simulink model "EvReferenceApplication"  (R2024a)
settings: Solver=daessc  StartTime=0  StopTime=2474  FixedStep=0.01  RelTol=1e-3
undefined symbols (not defined in the file or in its folder): anomaly_start, bat_temp_init, battery, driver_reaction, ext_wind, pipe, pump, pump_speed, radiator, sim_time, SRE, T_set, tank, valve
libraries: fl_lib x139, LiBatteryElements_lib x16, nesl_utility x14, SimscapeFluids_lib x7, autolibshared x2, simulink x1, autolibutils x1, slpidlib x1, simulink_extras x1
(part 3 of 4)

== system EvReferenceApplication/Passenger Car/Electric Plant/Powertrain Blockset/Motor ==
  MotTrqCmd : Inport
  MotSpd : Inport  Port=2
  BusVolt : Inport  Port=3
  MotGenEvDynamic : ModelReference  ModelNameDialog=MotGenEvDynamic.slx  SimulationMode=Normal  VariantControl=MotGenEvDynamic  ModelReferenceVersion=10.1
  MotGenEvMapped : ModelReference  ModelNameDialog=MotGenEvMapped.slx  SimulationMode=Normal  VariantControl=MotGenEvMapped  ModelReferenceVersion=8.3
  MotTrq : Outport  VectorParamsAs1DForOutWhenUnconnected=off
  MotCurnt : Outport  Port=2  VectorParamsAs1DForOutWhenUnconnected=off

== system EvReferenceApplication/Passenger Car/Electric Plant/Powertrain Blockset/Subsystem2 ==
  In Bus Element : Inport  PortName=BMS_Info  Element=SOC
  Bus Selector : BusSelector  OutputSignals=SOC_CC
  Data Type Conversion : DataTypeConversion  SaturateOnIntegerOverflow=off  RndMeth=Floor
  Rate Transition : RateTransition  Commented=through
  convert2percent : Gain  Gain=100
  BattSOC : Outport
  wires:
  In Bus Element/1 -> Bus Selector/1
  convert2percent/1 -> Data Type Conversion/1
  Bus Selector/1 -> convert2percent/1  "<SOC_CC>"
  Data Type Conversion/1 -> Rate Transition/1
  Rate Transition/1 -> BattSOC/1

== system EvReferenceApplication/Passenger Car/Electric Plant/Powertrain Blockset/Temp Selection ==
  AmbTmp : Inport
  Constant : Constant  Value=bat_temp_init
  Convert degC to K : Subsystem
  Manual Switch : ManualSwitch  CurrentSetting=0
  BattTmp : Outport
  wires:
  AmbTmp/1 -> Manual Switch/1
  Manual Switch/1 -> BattTmp/1
  Convert degC to K/1(Out1) -> Manual Switch/2
  Constant/1 -> Convert degC to K/1(In1)

== system EvReferenceApplication/Passenger Car/Electric Plant/Powertrain Blockset/BMS Signal Creation/Convert K to degC ==
  In1 : Inport
  Constant1 : Constant  Value=273.15
  Sum : Sum  Inputs=+-
  Out1 : Outport
  wires:
  In1/1 -> Sum/1
  Constant1/1 -> Sum/2
  Sum/1 -> Out1/1

== system EvReferenceApplication/Passenger Car/Electric Plant/Powertrain Blockset/Battery Cooling/Air Stream ==
  V : Inport
  Air density [kg/m^3] : Constant  Value=1.225
  Air velocity [m/s] : Bias  Bias=5  SaturateOnIntegerOverflow=off
  Product : Product  Inputs=3
  Radiator area [m^2] : Constant  Value=radiator.area_air
  Simulink-PS Converter1 : nesl_utility/Simulink-PS Converter  PhysicalDomain=network_engine_domain  SubClassName=ps_input  LeftPortType=input  RightPortType=output  PseudoPeriodic=off  Frequencies=[]  NoiseDistribution=none  NoiseParameters=[]  Unit=kg/s  AffineConversion=off  FilteringAndDerivatives=filter  SimscapeFilterOrder=1  InputFilterTimeConstant=0.01  UdotUserProvided=0
  mdot : PMIOPort  Side=Right
  wires:
  V/1 -> Air velocity [m/s]/1
  Product/1 -> Simulink-PS Converter1/1
  Radiator area [m^2]/1 -> Product/2
  Air density [kg/m^3]/1 -> Product/3
  Air velocity [m/s]/1 -> Product/1
  connections:
  mdot/RConn1 -- Simulink-PS Converter1/RConn1

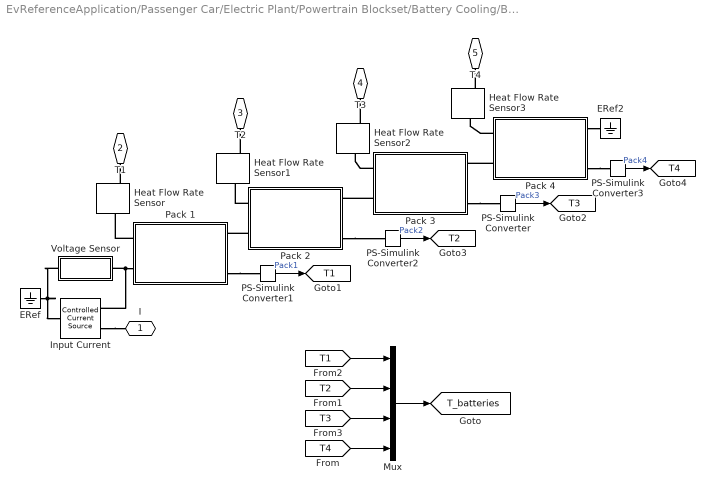
== system EvReferenceApplication/Passenger Car/Electric Plant/Powertrain Blockset/Battery Cooling/Battery1 ==
  ERef : fl_lib/Electrical/Electrical Elements/Electrical Reference
  ERef2 : fl_lib/Electrical/Electrical Elements/Electrical Reference
  Heat Flow Rate Sensor{,1..3} (4 alike) : fl_lib/Thermal/Thermal Sensors/Heat Flow Rate Sensor
  Input Current : fl_lib/Electrical/Electrical Sources/Controlled Current Source
  Mux : Mux
  PS-Simulink Converter{,1..3} (4 alike) : nesl_utility/PS-Simulink Converter  PhysicalDomain=network_engine_domain  SubClassName=ps_output  LeftPortType=input  RightPortType=output  PseudoPeriodic=off  Frequencies=[]  VectorFormat=1-D array  Unit=degC  AffineConversion=on
  Pack 1 : Subsystem  Tag=PublishSubsystem  mask(Lithium cell (one RC-branch equivalent circuit)){Ncells=battery.NCell, Qe_init=battery.Qe_init, T_init=bat_temp_init+273.15, Capacity_LUT=battery.capacity_LUT, Em_LUT=battery.Em_LUT, R0_LUT=battery.R0_LUT, R1_LUT=battery.R1_LUT, C1_LUT=battery.C1_LUT, cell_mass=battery.cell_mass, cell_Cp_heat=battery.cell_Cp, SOC_LUT=battery.SOC_LUT, Temperature_LUT=battery.temperature_LUT}
      mask prompts: Ncells "Number of series-connected cells"; Qe_init "Initial cell charge deficit (A*hr)"; T_init "Initial cell temperature (K)"; Capacity_LUT "Capacity (A*hr, 1xN table)"; Em_LUT "Em open-circuit voltage, Em (volts, MxN table)"; R0_LUT "R0 terminal resistance (ohms, MxN table)"; R1_LUT "R1 cell resistance (ohms, MxN table)"; C1_LUT "C1 capacitance (farads, MxN table)"; cell_mass "Cell mass (kg)"; cell_Cp_heat "Cell specific heat (J/kg/K)"; SOC_LUT "SOC table breakpoints (Mx1 array)"; Temperature_LUT "Temperature table breakpoints (K, 1xN array)"
      mask DialogControl ParameterTabVar0 Prompt: Main
      mask DialogControl ParameterTabVar01 Prompt: Electrical (per cell)
      mask DialogControl ParameterTabVar012 Prompt: Thermal (per cell)
      mask DialogControl ParameterTabVar0123 Prompt: Table Breakpoints
      mask Display:
      | % Battery icon
      | plot([2.5 1.3],[0 0])
      | plot([-0.6 -1.6 -1.6 -2.5],[0 0 -0.8 -0.8])
      | patch([1 1 -1 -1]*0.15+1.3,[-1 1 1 -1]*0.4,[0;0;0]);
      | patch([1 1 -1 -1]*0.15+0.0,[-1 1 1 -1]*0.4,[0;0;0]);
      | patch([1 1 -1 -1]*0.15+0.7,[-1 1 1 -1]*0.8,[0;0;0]);
      | patch([1 1 -1 -1]*0.15-0.6,[-1 1 1 -1]*0.8,[0;0;0]);
      | % Thermal port
      | plot([-1.6,-1.3],[1.2,1.2])
      | plot([-1.6,-1.3],[0.5,0.5])
      | plot([-1.6,-2.5],[0.8,0.8])
      | plot(0.2*sin(0:2*pi/50:2*pi)-1.6,0.35*cos(0:2*pi/50:2*pi)+0.85)
      | plot(0.2*sin(0:2*pi/50:pi)-1.3,0.35*cos(0:2*pi/50:pi)+0.85)
      | 
      | % Plot points to set plot range
      | color('white');plot(2.5,1.5);plot(-2.5,-1.5)
      | 
      | color('red')
      | port_label('LConn',1,'H')
      | port_label('LConn',2,'+')
      | port_label('RConn',1,'-')
      | port_label('RConn',2,'SOC')
      | port_label('RConn',3,'T')
  Pack 2 : Subsystem  Tag=PublishSubsystem  mask(Lithium cell (one RC-branch equivalent circuit)){Ncells=battery.NCell, Qe_init=battery.Qe_init, T_init=bat_temp_init+273.15, Capacity_LUT=battery.capacity_LUT, Em_LUT=battery.Em_LUT, R0_LUT=battery.R0_LUT, R1_LUT=battery.R1_LUT, C1_LUT=battery.C1_LUT, cell_mass=battery.cell_mass, cell_Cp_heat=battery.cell_Cp, SOC_LUT=battery.SOC_LUT, Temperature_LUT=battery.temperature_LUT}
      mask prompts: Ncells "Number of series-connected cells"; Qe_init "Initial cell charge deficit (A*hr)"; T_init "Initial cell temperature (K)"; Capacity_LUT "Capacity (A*hr, 1xN table)"; Em_LUT "Em open-circuit voltage, Em (volts, MxN table)"; R0_LUT "R0 terminal resistance (ohms, MxN table)"; R1_LUT "R1 cell resistance (ohms, MxN table)"; C1_LUT "C1 capacitance (farads, MxN table)"; cell_mass "Cell mass (kg)"; cell_Cp_heat "Cell specific heat (J/kg/K)"; SOC_LUT "SOC table breakpoints (Mx1 array)"; Temperature_LUT "Temperature table breakpoints (K, 1xN array)"
      mask DialogControl ParameterTabVar0 Prompt: Main
      mask DialogControl ParameterTabVar01 Prompt: Electrical (per cell)
      mask DialogControl ParameterTabVar012 Prompt: Thermal (per cell)
      mask DialogControl ParameterTabVar0123 Prompt: Table Breakpoints
      mask Display:
      | % Battery icon
      | plot([2.5 1.3],[0 0])
      | plot([-0.6 -1.6 -1.6 -2.5],[0 0 -0.8 -0.8])
      | patch([1 1 -1 -1]*0.15+1.3,[-1 1 1 -1]*0.4,[0;0;0]);
      | patch([1 1 -1 -1]*0.15+0.0,[-1 1 1 -1]*0.4,[0;0;0]);
      | patch([1 1 -1 -1]*0.15+0.7,[-1 1 1 -1]*0.8,[0;0;0]);
      | patch([1 1 -1 -1]*0.15-0.6,[-1 1 1 -1]*0.8,[0;0;0]);
      | % Thermal port
      | plot([-1.6,-1.3],[1.2,1.2])
      | plot([-1.6,-1.3],[0.5,0.5])
      | plot([-1.6,-2.5],[0.8,0.8])
      | plot(0.2*sin(0:2*pi/50:2*pi)-1.6,0.35*cos(0:2*pi/50:2*pi)+0.85)
      | plot(0.2*sin(0:2*pi/50:pi)-1.3,0.35*cos(0:2*pi/50:pi)+0.85)
      | 
      | % Plot points to set plot range
      | color('white');plot(2.5,1.5);plot(-2.5,-1.5)
      | 
      | color('red')
      | port_label('LConn',1,'H')
      | port_label('LConn',2,'+')
      | port_label('RConn',1,'-')
      | port_label('RConn',2,'SOC')
      | port_label('RConn',3,'T')
  Pack 3 : Subsystem  Tag=PublishSubsystem  mask(Lithium cell (one RC-branch equivalent circuit)){Ncells=battery.NCell, Qe_init=battery.Qe_init, T_init=bat_temp_init+273.15, Capacity_LUT=battery.capacity_LUT, Em_LUT=battery.Em_LUT, R0_LUT=battery.R0_LUT, R1_LUT=battery.R1_LUT, C1_LUT=battery.C1_LUT, cell_mass=battery.cell_mass, cell_Cp_heat=battery.cell_Cp, SOC_LUT=battery.SOC_LUT, Temperature_LUT=battery.temperature_LUT}
      mask prompts: Ncells "Number of series-connected cells"; Qe_init "Initial cell charge deficit (A*hr)"; T_init "Initial cell temperature (K)"; Capacity_LUT "Capacity (A*hr, 1xN table)"; Em_LUT "Em open-circuit voltage, Em (volts, MxN table)"; R0_LUT "R0 terminal resistance (ohms, MxN table)"; R1_LUT "R1 cell resistance (ohms, MxN table)"; C1_LUT "C1 capacitance (farads, MxN table)"; cell_mass "Cell mass (kg)"; cell_Cp_heat "Cell specific heat (J/kg/K)"; SOC_LUT "SOC table breakpoints (Mx1 array)"; Temperature_LUT "Temperature table breakpoints (K, 1xN array)"
      mask DialogControl ParameterTabVar0 Prompt: Main
      mask DialogControl ParameterTabVar01 Prompt: Electrical (per cell)
      mask DialogControl ParameterTabVar012 Prompt: Thermal (per cell)
      mask DialogControl ParameterTabVar0123 Prompt: Table Breakpoints
      mask Display:
      | % Battery icon
      | plot([2.5 1.3],[0 0])
      | plot([-0.6 -1.6 -1.6 -2.5],[0 0 -0.8 -0.8])
      | patch([1 1 -1 -1]*0.15+1.3,[-1 1 1 -1]*0.4,[0;0;0]);
      | patch([1 1 -1 -1]*0.15+0.0,[-1 1 1 -1]*0.4,[0;0;0]);
      | patch([1 1 -1 -1]*0.15+0.7,[-1 1 1 -1]*0.8,[0;0;0]);
      | patch([1 1 -1 -1]*0.15-0.6,[-1 1 1 -1]*0.8,[0;0;0]);
      | % Thermal port
      | plot([-1.6,-1.3],[1.2,1.2])
      | plot([-1.6,-1.3],[0.5,0.5])
      | plot([-1.6,-2.5],[0.8,0.8])
      | plot(0.2*sin(0:2*pi/50:2*pi)-1.6,0.35*cos(0:2*pi/50:2*pi)+0.85)
      | plot(0.2*sin(0:2*pi/50:pi)-1.3,0.35*cos(0:2*pi/50:pi)+0.85)
      | 
      | % Plot points to set plot range
      | color('white');plot(2.5,1.5);plot(-2.5,-1.5)
      | 
      | color('red')
      | port_label('LConn',1,'H')
      | port_label('LConn',2,'+')
      | port_label('RConn',1,'-')
      | port_label('RConn',2,'SOC')
      | port_label('RConn',3,'T')
  Pack 4 : Subsystem  Tag=PublishSubsystem  mask(Lithium cell (one RC-branch equivalent circuit)){Ncells=battery.NCell, Qe_init=battery.Qe_init, T_init=bat_temp_init+273.15, Capacity_LUT=battery.capacity_LUT, Em_LUT=battery.Em_LUT, R0_LUT=battery.R0_LUT, R1_LUT=battery.R1_LUT, C1_LUT=battery.C1_LUT, cell_mass=battery.cell_mass, cell_Cp_heat=battery.cell_Cp, SOC_LUT=battery.SOC_LUT, Temperature_LUT=battery.temperature_LUT}
      mask prompts: Ncells "Number of series-connected cells"; Qe_init "Initial cell charge deficit (A*hr)"; T_init "Initial cell temperature (K)"; Capacity_LUT "Capacity (A*hr, 1xN table)"; Em_LUT "Em open-circuit voltage, Em (volts, MxN table)"; R0_LUT "R0 terminal resistance (ohms, MxN table)"; R1_LUT "R1 cell resistance (ohms, MxN table)"; C1_LUT "C1 capacitance (farads, MxN table)"; cell_mass "Cell mass (kg)"; cell_Cp_heat "Cell specific heat (J/kg/K)"; SOC_LUT "SOC table breakpoints (Mx1 array)"; Temperature_LUT "Temperature table breakpoints (K, 1xN array)"
      mask DialogControl ParameterTabVar0 Prompt: Main
      mask DialogControl ParameterTabVar01 Prompt: Electrical (per cell)
      mask DialogControl ParameterTabVar012 Prompt: Thermal (per cell)
      mask DialogControl ParameterTabVar0123 Prompt: Table Breakpoints
      mask Display:
      | % Battery icon
      | plot([2.5 1.3],[0 0])
      | plot([-0.6 -1.6 -1.6 -2.5],[0 0 -0.8 -0.8])
      | patch([1 1 -1 -1]*0.15+1.3,[-1 1 1 -1]*0.4,[0;0;0]);
      | patch([1 1 -1 -1]*0.15+0.0,[-1 1 1 -1]*0.4,[0;0;0]);
      | patch([1 1 -1 -1]*0.15+0.7,[-1 1 1 -1]*0.8,[0;0;0]);
      | patch([1 1 -1 -1]*0.15-0.6,[-1 1 1 -1]*0.8,[0;0;0]);
      | % Thermal port
      | plot([-1.6,-1.3],[1.2,1.2])
      | plot([-1.6,-1.3],[0.5,0.5])
      | plot([-1.6,-2.5],[0.8,0.8])
      | plot(0.2*sin(0:2*pi/50:2*pi)-1.6,0.35*cos(0:2*pi/50:2*pi)+0.85)
      | plot(0.2*sin(0:2*pi/50:pi)-1.3,0.35*cos(0:2*pi/50:pi)+0.85)
      | 
      | % Plot points to set plot range
      | color('white');plot(2.5,1.5);plot(-2.5,-1.5)
      | 
      | color('red')
      | port_label('LConn',1,'H')
      | port_label('LConn',2,'+')
      | port_label('RConn',1,'-')
      | port_label('RConn',2,'SOC')
      | port_label('RConn',3,'T')
  Voltage Sensor : Subsystem
      mask Display: disp('V_load')
  I : PMIOPort  Side=Left
  T1 : PMIOPort  Port=2  Side=Right
  T2 : PMIOPort  Port=3  Side=Right
  T3 : PMIOPort  Port=4  Side=Right
  T4 : PMIOPort  Port=5  Side=Right
  tag scope: T1=global, T2=global, T3=global, T4=global, T_batteries=global
  wires:
  PS-Simulink Converter/1 -> [T3]  "Pack3"
  PS-Simulink Converter2/1 -> [T2]  "Pack2"
  PS-Simulink Converter3/1 -> [T4]  "Pack4"
  [T1] -> Mux/1
  [T2] -> Mux/2
  [T3] -> Mux/3
  [T4] -> Mux/4
  Mux/1 -> [T_batteries]
  PS-Simulink Converter1/1 -> [T1]  "Pack1"
  connections:
  Pack 3/LConn2 -- Pack 2/RConn1
  Pack 3/RConn3 -- PS-Simulink Converter/LConn1
  Voltage Sensor/LConn1 -- Pack 1/LConn2 -- Input Current/RConn2
  Pack 2/LConn2 -- Pack 1/RConn1
  Pack 4/RConn1 -- ERef2/LConn1
  Input Current/RConn1 -- I/RConn1
  Voltage Sensor/RConn1 -- ERef/LConn1 -- Input Current/LConn1
  Pack 4/LConn2 -- Pack 3/RConn1
  Pack 2/RConn3 -- PS-Simulink Converter2/LConn1
  Pack 4/RConn3 -- PS-Simulink Converter3/LConn1
  Pack 1/RConn3 -- PS-Simulink Converter1/LConn1
  Pack 1/LConn1 -- Heat Flow Rate Sensor/LConn1
  Heat Flow Rate Sensor/RConn2 -- T1/RConn1
  Heat Flow Rate Sensor1/RConn2 -- T2/RConn1
  Pack 2/LConn1 -- Heat Flow Rate Sensor1/LConn1
  Heat Flow Rate Sensor2/RConn2 -- T3/RConn1
  Pack 3/LConn1 -- Heat Flow Rate Sensor2/LConn1
  Heat Flow Rate Sensor3/RConn2 -- T4/RConn1
  Pack 4/LConn1 -- Heat Flow Rate Sensor3/LConn1

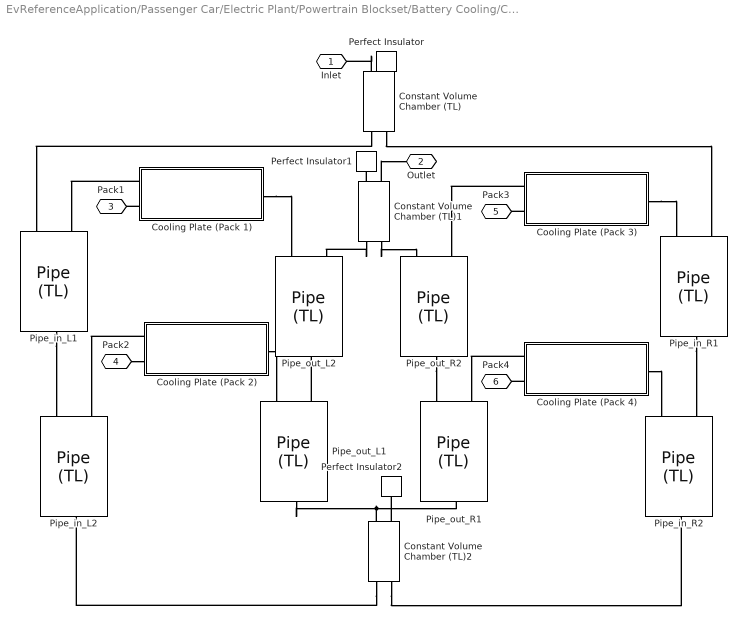
== system EvReferenceApplication/Passenger Car/Electric Plant/Powertrain Blockset/Battery Cooling/Cold Plate ==
  Constant Volume Chamber (TL) : fl_lib/Thermal Liquid/Elements/Constant Volume Chamber (TL)  volume=0.001 m^3  num_ports=foundation.enum.num_ports.three  area_A=3 cm^2  area_B=3 cm^2  area_C=3 cm^2  area_D=0.01 m^2  p_I_specify=off  p_I_priority=High  p_I=0.101325 MPa  p_I_nominal_specify=off  p_I_nominal_unit=MPa  p_I_nominal_value=1  T_I_specify=on  T_I_priority=High  T_I=bat_temp_init+273.15 K  T_I_nominal_specify=off  T_I_nominal_unit=K  T_I_nominal_value=1  u_I_specify=off  u_I_priority=None  u_I=83.90600000000001 kJ/kg  u_I_nominal_specify=off  u_I_nominal_unit=kJ/kg  u_I_nominal_value=1  rho_I_specify=off  rho_I_priority=None  rho_I=998.21 kg/m^3  rho_I_nominal_specify=off  rho_I_nominal_unit=kg/m^3  rho_I_nominal_value=1
      settings: InternalSimscapePortConfiguration="{\"Bottom\":[],\"Left\":[{\"id\":\"A\",\"label\":\"A\",\"type\":\"foundation.thermal_liquid.thermal_liquid\"},{\"id\":\"H\",\"label\":\"H\",\"type\":\"foundation.thermal.thermal\"}],\"Right\":[{\"id\":\"B\",\"label\":\"B\",\"type\":\"foundation.thermal_liquid.thermal_liquid\"},{\"id\":\"C\",\"label\":\"C\",\"type\":\"foundation.thermal_liquid.thermal_liquid\"}],\"Top\":[]}"
  Constant Volume Chamber (TL)1 : fl_lib/Thermal Liquid/Elements/Constant Volume Chamber (TL)  volume=0.001 m^3  num_ports=foundation.enum.num_ports.three  area_A=3 cm^2  area_B=3 cm^2  area_C=3 cm^2  area_D=0.01 m^2  p_I_specify=off  p_I_priority=High  p_I=0.101325 MPa  p_I_nominal_specify=off  p_I_nominal_unit=MPa  p_I_nominal_value=1  T_I_specify=on  T_I_priority=High  T_I=bat_temp_init+273.15 K  T_I_nominal_specify=off  T_I_nominal_unit=K  T_I_nominal_value=1  u_I_specify=off  u_I_priority=None  u_I=83.90600000000001 kJ/kg  u_I_nominal_specify=off  u_I_nominal_unit=kJ/kg  u_I_nominal_value=1  rho_I_specify=off  rho_I_priority=None  rho_I=998.21 kg/m^3  rho_I_nominal_specify=off  rho_I_nominal_unit=kg/m^3  rho_I_nominal_value=1
      settings: InternalSimscapePortConfiguration="{\"Bottom\":[],\"Left\":[{\"id\":\"A\",\"label\":\"A\",\"type\":\"foundation.thermal_liquid.thermal_liquid\"},{\"id\":\"H\",\"label\":\"H\",\"type\":\"foundation.thermal.thermal\"}],\"Right\":[{\"id\":\"B\",\"label\":\"B\",\"type\":\"foundation.thermal_liquid.thermal_liquid\"},{\"id\":\"C\",\"label\":\"C\",\"type\":\"foundation.thermal_liquid.thermal_liquid\"}],\"Top\":[]}"
  Constant Volume Chamber (TL)2 : fl_lib/Thermal Liquid/Elements/Constant Volume Chamber (TL)  volume=0.001 m^3  num_ports=foundation.enum.num_ports.three  area_A=3 cm^2  area_B=3 cm^2  area_C=3 cm^2  area_D=0.01 m^2  p_I_specify=off  p_I_priority=High  p_I=0.101325 MPa  p_I_nominal_specify=off  p_I_nominal_unit=MPa  p_I_nominal_value=1  T_I_specify=on  T_I_priority=High  T_I=bat_temp_init+273.15 K  T_I_nominal_specify=off  T_I_nominal_unit=K  T_I_nominal_value=1  u_I_specify=off  u_I_priority=None  u_I=83.90600000000001 kJ/kg  u_I_nominal_specify=off  u_I_nominal_unit=kJ/kg  u_I_nominal_value=1  rho_I_specify=off  rho_I_priority=None  rho_I=998.21 kg/m^3  rho_I_nominal_specify=off  rho_I_nominal_unit=kg/m^3  rho_I_nominal_value=1
      settings: InternalSimscapePortConfiguration="{\"Bottom\":[],\"Left\":[{\"id\":\"A\",\"label\":\"A\",\"type\":\"foundation.thermal_liquid.thermal_liquid\"},{\"id\":\"H\",\"label\":\"H\",\"type\":\"foundation.thermal.thermal\"}],\"Right\":[{\"id\":\"B\",\"label\":\"B\",\"type\":\"foundation.thermal_liquid.thermal_liquid\"},{\"id\":\"C\",\"label\":\"C\",\"type\":\"foundation.thermal_liquid.thermal_liquid\"}],\"Top\":[]}"
  Cooling Plate (Pack 1) : Subsystem
  Cooling Plate (Pack 2) : Subsystem
  Cooling Plate (Pack 3) : Subsystem
  Cooling Plate (Pack 4) : Subsystem
  Perfect Insulator : fl_lib/Thermal/Thermal Elements/Perfect Insulator  T_specify=off  T_priority=None  T=0 K  T_nominal_specify=off  T_nominal_unit=K  T_nominal_value=1
  Perfect Insulator1 : fl_lib/Thermal/Thermal Elements/Perfect Insulator  T_specify=off  T_priority=None  T=0 K  T_nominal_specify=off  T_nominal_unit=K  T_nominal_value=1
  Perfect Insulator2 : fl_lib/Thermal/Thermal Elements/Perfect Insulator  T_specify=off  T_priority=None  T=0 K  T_nominal_specify=off  T_nominal_unit=K  T_nominal_value=1
  Pipe_in_L1 : fl_lib/Thermal Liquid/Elements/Pipe (TL)  length=1.5 m  area=3 cm^2  Dh=0.92 cm  length_add=0 m  roughness=15e-6 m  Re_lam=2000  Re_tur=4000  shape_factor=64  Nu_lam=3.66  dynamic_compressibility=simscape.enum.onoff.on  inertia=simscape.enum.onoff.off  p0=0.101325 MPa  T0=bat_temp_init+273.15 K  mdot0=0 kg/s
  Pipe_in_L2 : fl_lib/Thermal Liquid/Elements/Pipe (TL)  length=1.5 m  area=3 cm^2  Dh=0.92 cm  length_add=0 m  roughness=15e-6 m  Re_lam=2000  Re_tur=4000  shape_factor=64  Nu_lam=3.66  dynamic_compressibility=simscape.enum.onoff.on  inertia=simscape.enum.onoff.off  p0=0.101325 MPa  T0=bat_temp_init+273.15 K  mdot0=0 kg/s
  Pipe_in_R1 : fl_lib/Thermal Liquid/Elements/Pipe (TL)  length=1.5 m  area=3 cm^2  Dh=0.92 cm  length_add=0 m  roughness=15e-6 m  Re_lam=2000  Re_tur=4000  shape_factor=64  Nu_lam=3.66  dynamic_compressibility=simscape.enum.onoff.on  inertia=simscape.enum.onoff.off  p0=0.101325 MPa  T0=bat_temp_init+273.15 K  mdot0=0 kg/s
  Pipe_in_R2 : fl_lib/Thermal Liquid/Elements/Pipe (TL)  length=1.5 m  area=3 cm^2  Dh=0.92 cm  length_add=0 m  roughness=15e-6 m  Re_lam=2000  Re_tur=4000  shape_factor=64  Nu_lam=3.66  dynamic_compressibility=simscape.enum.onoff.on  inertia=simscape.enum.onoff.off  p0=0.101325 MPa  T0=bat_temp_init+273.15 K  mdot0=0 kg/s
  Pipe_out_L1 : fl_lib/Thermal Liquid/Elements/Pipe (TL)  length=1 m  area=3 cm^2  Dh=0.92 cm  length_add=0 m  roughness=15e-6 m  Re_lam=2000  Re_tur=4000  shape_factor=64  Nu_lam=3.66  dynamic_compressibility=simscape.enum.onoff.on  inertia=simscape.enum.onoff.off  p0=0.101325 MPa  T0=bat_temp_init+273.15 K  mdot0=0 kg/s
  Pipe_out_L2 : fl_lib/Thermal Liquid/Elements/Pipe (TL)  length=1 m  area=3 cm^2  Dh=0.92 cm  length_add=0 m  roughness=15e-6 m  Re_lam=2000  Re_tur=4000  shape_factor=64  Nu_lam=3.66  dynamic_compressibility=simscape.enum.onoff.on  inertia=simscape.enum.onoff.off  p0=0.101325 MPa  T0=bat_temp_init+273.15 K  mdot0=0 kg/s
      settings: LogSimulationData=on
  Pipe_out_R1 : fl_lib/Thermal Liquid/Elements/Pipe (TL)  length=1 m  area=3 cm^2  Dh=0.92 cm  length_add=0 m  roughness=15e-6 m  Re_lam=2000  Re_tur=4000  shape_factor=64  Nu_lam=3.66  dynamic_compressibility=simscape.enum.onoff.on  inertia=simscape.enum.onoff.off  p0=0.101325 MPa  T0=bat_temp_init+273.15 K  mdot0=0 kg/s
  Pipe_out_R2 : fl_lib/Thermal Liquid/Elements/Pipe (TL)  length=1 m  area=3 cm^2  Dh=0.92 cm  length_add=0 m  roughness=15e-6 m  Re_lam=2000  Re_tur=4000  shape_factor=64  Nu_lam=3.66  dynamic_compressibility=simscape.enum.onoff.on  inertia=simscape.enum.onoff.off  p0=0.101325 MPa  T0=bat_temp_init+273.15 K  mdot0=0 kg/s
  Inlet : PMIOPort  Side=Left
  Outlet : PMIOPort  Port=2  Side=Left
  Pack1 : PMIOPort  Port=3  Side=Right
  Pack2 : PMIOPort  Port=4  Side=Right
  Pack3 : PMIOPort  Port=5  Side=Right
  Pack4 : PMIOPort  Port=6  Side=Right
  connections:
  Constant Volume Chamber (TL)/LConn1 -- Inlet/RConn1
  Constant Volume Chamber (TL)/LConn2 -- Perfect Insulator/LConn1
  Constant Volume Chamber (TL)/RConn1 -- Pipe_in_L1/LConn1
  Pipe_in_R1/RConn1 -- Pipe_in_R2/LConn1
  Constant Volume Chamber (TL)1/LConn2 -- Perfect Insulator1/LConn1
  Pipe_out_L1/LConn1 -- Pipe_out_L2/RConn1
  Pipe_out_R2/RConn1 -- Pipe_out_R1/LConn1
  Constant Volume Chamber (TL)1/LConn1 -- Outlet/RConn1
  Cooling Plate (Pack 3)/LConn1 -- Pipe_out_R2/LConn2
  Cooling Plate (Pack 1)/LConn1 -- Pipe_in_L1/LConn2
  Cooling Plate (Pack 1)/RConn1 -- Pipe_out_L2/LConn2
  Cooling Plate (Pack 2)/RConn1 -- Pipe_out_L1/LConn2
  Cooling Plate (Pack 2)/LConn1 -- Pipe_in_L2/LConn2
  Pipe_in_L1/RConn1 -- Pipe_in_L2/LConn1
  Constant Volume Chamber (TL)1/RConn1 -- Pipe_out_R2/LConn1
  Cooling Plate (Pack 3)/RConn1 -- Pipe_in_R1/LConn2
  Constant Volume Chamber (TL)2/RConn1 -- Pipe_in_L2/RConn1
  Cooling Plate (Pack 4)/RConn1 -- Pipe_in_R2/LConn2
  Cooling Plate (Pack 4)/LConn1 -- Pipe_out_R1/LConn2
  Constant Volume Chamber (TL)2/RConn2 -- Pipe_in_R2/RConn1
  Cooling Plate (Pack 1)/LConn2 -- Pack1/RConn1
  Pack2/RConn1 -- Cooling Plate (Pack 2)/LConn2
  Cooling Plate (Pack 3)/LConn2 -- Pack3/RConn1
  Cooling Plate (Pack 4)/LConn2 -- Pack4/RConn1
  Constant Volume Chamber (TL)1/RConn2 -- Pipe_out_L2/LConn1
  Constant Volume Chamber (TL)2/LConn2 -- Perfect Insulator2/LConn1
  Pipe_out_L1/RConn1 -- Pipe_out_R1/RConn1 -- Constant Volume Chamber (TL)2/LConn1
  Constant Volume Chamber (TL)/RConn2 -- Pipe_in_R1/LConn1

== system EvReferenceApplication/Passenger Car/Electric Plant/Powertrain Blockset/Battery Cooling/Controller ==
  T_set : Inport
  Ideal Angular Velocity Source : fl_lib/Mechanical/Mechanical Sources/Ideal Angular Velocity Source
  Mechanical Rotational Reference : fl_lib/Mechanical/Rotational Elements/Mechanical Rotational Reference
  Product : Product
  Pump response delay : TransferFcn  Denominator=[20 1]
  Pump speed [rpm] : Constant  Value=pump.omega
  Relay : Relay  OnSwitchValue=+1  OffSwitchValue=0.1
  Sensors : Subsystem
  Simulink-PS Converter1 : nesl_utility/Simulink-PS Converter  PhysicalDomain=network_engine_domain  SubClassName=ps_input  LeftPortType=input  RightPortType=output  PseudoPeriodic=off  Frequencies=[]  NoiseDistribution=none  NoiseParameters=[]  Unit=rpm  AffineConversion=off  FilteringAndDerivatives=provide  SimscapeFilterOrder=1  InputFilterTimeConstant=0.001  UdotUserProvided=0
  Sum : Sum  Inputs=|-+
  R : PMIOPort  Side=Right
  wires:
  T_set/1 -> Sum/1
  Pump speed [rpm]/1 -> Product/1
  [T3] -> Sum/2
  Sum/1 -> Relay/1
  Relay/1 -> Product/2
  Product/1 -> Pump response delay/1
  Pump response delay/1 -> Simulink-PS Converter1/1
  connections:
  Sensors/RConn1 -- R/RConn1
  Ideal Angular Velocity Source/RConn2 -- Mechanical Rotational Reference/LConn1
  Simulink-PS Converter1/RConn1 -- Ideal Angular Velocity Source/RConn1
  Sensors/LConn1 -- Ideal Angular Velocity Source/LConn1

== system EvReferenceApplication/Passenger Car/Electric Plant/Powertrain Blockset/Battery Cooling/Environment ==
  Convective Heat Transfer : fl_lib/Thermal/Thermal Elements/Convective Heat Transfer  thermal_type=foundation.enum.constant_variable.constant  area=tank.area_wall/2 m^2  heat_tr_coeff=20 W/(m^2 * K)  min_heat_tr_coeff=1e-3 W/(K*m^2)  T_specify=off  T_priority=None  T=0 K  T_nominal_specify=off  T_nominal_unit=K  T_nominal_value=1  Q_specify=off  Q_priority=None  Q=0 W  Q_nominal_specify=off  Q_nominal_unit=W  Q_nominal_value=1
  Convective Heat Transfer1 : fl_lib/Thermal/Thermal Elements/Convective Heat Transfer  thermal_type=foundation.enum.constant_variable.constant  area=tank.area_wall/2 m^2  heat_tr_coeff=20 W/(m^2 * K)  min_heat_tr_coeff=1e-3 W/(K*m^2)  T_specify=off  T_priority=None  T=0 K  T_nominal_specify=off  T_nominal_unit=K  T_nominal_value=1  Q_specify=off  Q_priority=None  Q=0 W  Q_nominal_specify=off  Q_nominal_unit=W  Q_nominal_value=1
  T_ambient : fl_lib/Thermal/Thermal Sources/Temperature Source  temperature=bat_temp_init degC
  T_ambient1 : fl_lib/Thermal/Thermal Sources/Temperature Source  temperature=bat_temp_init degC
  TH1 : PMIOPort  Side=Left
  TH2 : PMIOPort  Port=2  Side=Left
  connections:
  T_ambient1/LConn1 -- Convective Heat Transfer1/RConn1
  Convective Heat Transfer/RConn1 -- T_ambient/LConn1
  Convective Heat Transfer1/LConn1 -- TH2/RConn1
  Convective Heat Transfer/LConn1 -- TH1/RConn1

== system EvReferenceApplication/Passenger Car/Electric Plant/Powertrain Blockset/Battery Cooling/Heating-Cooling Unit ==
  4 Way Valve : Subsystem
  Constant Volume Chamber (TL) : fl_lib/Thermal Liquid/Elements/Constant Volume Chamber (TL)  volume=5 cm^3  num_ports=foundation.enum.num_ports.four  area_A=pipe.area m^2  area_B=pipe.area*10 m^2  area_C=pipe.area m^2  area_D=pipe.area m^2  p_I_specify=off  p_I_priority=High  p_I=0.101325 MPa  p_I_nominal_specify=off  p_I_nominal_unit=MPa  p_I_nominal_value=1  T_I_specify=on  T_I_priority=High  T_I=bat_temp_init+273.15 K  T_I_nominal_specify=off  T_I_nominal_unit=K  T_I_nominal_value=1  u_I_specify=off  u_I_priority=None  u_I=83.90600000000001 kJ/kg  u_I_nominal_specify=off  u_I_nominal_unit=kJ/kg  u_I_nominal_value=1  rho_I_specify=off  rho_I_priority=None  rho_I=998.21 kg/m^3  rho_I_nominal_specify=off  rho_I_nominal_unit=kg/m^3  rho_I_nominal_value=1
      settings: InternalSimscapePortConfiguration="{\"Bottom\":[],\"Left\":[{\"id\":\"A\",\"label\":\"A\",\"type\":\"foundation.thermal_liquid.thermal_liquid\"},{\"id\":\"H\",\"label\":\"H\",\"type\":\"foundation.thermal.thermal\"}],\"Right\":[{\"id\":\"B\",\"label\":\"B\",\"type\":\"foundation.thermal_liquid.thermal_liquid\"},{\"id\":\"C\",\"label\":\"C\",\"type\":\"foundation.thermal_liquid.thermal_liquid\"},{\"id\":\"D\",\"label\":\"D\",\"type\":\"foundation.thermal_liquid.thermal_liquid\"}],\"Top\":[]}"
  Controller : Subsystem
  Coolant temperature : Subsystem
  Cooling Inlet : fl_lib/Thermal Liquid/Elements/Pipe (TL)  length=0.75 m  area=pipe.area cm^2  Dh=pipe.Dh cm  length_add=0 m  roughness=15e-6 m  Re_lam=2000  Re_tur=4000  shape_factor=64  Nu_lam=3.66  dynamic_compressibility=simscape.enum.onoff.on  inertia=simscape.enum.onoff.off  p0=0.101325 MPa  T0=bat_temp_init+273.15 K  mdot0=0 kg/s
  Heater : Subsystem
  Perfect Insulator : fl_lib/Thermal/Thermal Elements/Perfect Insulator  T_specify=off  T_priority=None  T=0 K  T_nominal_specify=off  T_nominal_unit=K  T_nominal_value=1
  Perfect Insulator3 : fl_lib/Thermal/Thermal Elements/Perfect Insulator  T_specify=off  T_priority=None  T=0 K  T_nominal_specify=off  T_nominal_unit=K  T_nominal_value=1
  Radiator : Subsystem
  Refrigerant System : Subsystem
  B1 : PMIOPort  Side=Right
  A1 : PMIOPort  Port=2  Side=Left
  B2 : PMIOPort  Port=3  Side=Left
  A2 : PMIOPort  Port=4  Side=Right
  wires:
  Coolant temperature/1(T) -> Controller/1(T)
  connections:
  Constant Volume Chamber (TL)/RConn1 -- Refrigerant System/LConn1
  4 Way Valve/RConn2 -- Controller/RConn1
  4 Way Valve/LConn2 -- Radiator/RConn2
  4 Way Valve/RConn1 -- Cooling Inlet/RConn1
  Perfect Insulator3/LConn1 -- Cooling Inlet/LConn2
  Cooling Inlet/LConn1 -- A2/RConn1
  Radiator/RConn1 -- A1/RConn1
  4 Way Valve/LConn1 -- Refrigerant System/RConn1
  Radiator/LConn1 -- B1/RConn1
  Constant Volume Chamber (TL)/RConn3 -- Heater/LConn1
  Constant Volume Chamber (TL)/LConn1 -- Coolant temperature/LConn1 -- B2/RConn1
  4 Way Valve/LConn3 -- Heater/RConn1
  Constant Volume Chamber (TL)/RConn2 -- Radiator/LConn2
  Perfect Insulator/LConn1 -- Constant Volume Chamber (TL)/LConn2

== system EvReferenceApplication/Passenger Car/Electric Plant/Powertrain Blockset/Battery Cooling/Pump Power ==
  Product : Product
  kW : Gain  Gain=1e-3
  Pump power [W] : Outport  VectorParamsAs1DForOutWhenUnconnected=off
  wires:
  [torque] -> Product/1
  [omega] -> Product/2
  Product/1 -> kW/1
  kW/1 -> Pump power [W]/1

== system EvReferenceApplication/Passenger Car/Electric Plant/Powertrain Blockset/Battery Cooling/Subsystem1 ==
  Mux : Mux  Inputs=3
  T_max : Constant  Commented=on  Value=T_set + 1
  T_min : Constant  Commented=on  Value=T_set - 0.5
  Out1 : Outport  VectorParamsAs1DForOutWhenUnconnected=off
  wires:
  T_max/1 -> Mux/2
  T_min/1 -> Mux/3
  [T_batteries] -> Mux/1
  Mux/1 -> Out1/1

== system EvReferenceApplication/Passenger Car/Electric Plant/Powertrain Blockset/Temp Selection/Convert degC to K ==
  In1 : Inport
  Constant1 : Constant  Value=273.15
  Sum : Sum
  Out1 : Outport
  wires:
  In1/1 -> Sum/1
  Constant1/1 -> Sum/2
  Sum/1 -> Out1/1

== system EvReferenceApplication/Passenger Car/Electric Plant/Powertrain Blockset/Battery Cooling/Battery1/Pack 1 ==
  note: Scale up voltage drop
      | to total of N cells
  Controlled Voltage Source : fl_lib/Electrical/Electrical Sources/Controlled Voltage Source
  Lithium Cell 1RC : Subsystem  Tag=PublishSubsystem
      mask Display:
      | % Battery icon
      | plot([0 0 0.8 0.8],[0.2 0.9 0.9 1.5])
      | plot([0 0 0.8 0.8],-[0.2 0.9 0.9 1.5])
      | patch([-0.4 0.4 0.4 -0.4],[-0.45 -0.45 -0.15 -0.15],[0;0;0]);
      | patch([-0.9 0.9 0.9 -0.9],[0.15 0.15 0.45 0.45],[0;0;0]);
      | 
      | % Plot points to set plot range
      | color('white');plot(1.5,1.5);plot(-1.5,-1.5)
      | 
      | color('red')
      | port_label('RConn',1,'P')
      | port_label('RConn',2,'+')
      | port_label('LConn',1,'T')
      | port_label('LConn',2,'-')
  N : fl_lib/Physical Signals/Functions/PS Gain  gain=Ncells
  N-1 : fl_lib/Physical Signals/Functions/PS Gain  gain=(Ncells-1)
  Thermal Model : Subsystem
  Voltage Sensor : fl_lib/Electrical/Electrical Sensors/Voltage Sensor
  - : PMIOPort  Tag=PMCPort  Side=Right
  H : PMIOPort  Tag=PMCPort  Port=2  Side=Left
  + : PMIOPort  Tag=PMCPort  Port=3  Side=Left
  SOC : PMIOPort  Port=4  Side=Right
  T : PMIOPort  Port=5  Side=Right
  connections:
  SOC/RConn1 -- Lithium Cell 1RC/RConn2
  N/RConn1 -- Thermal Model/LConn2
  N/LConn1 -- Lithium Cell 1RC/RConn1
  Lithium Cell 1RC/LConn1 -- T/RConn1 -- Thermal Model/RConn1
  Thermal Model/LConn1 -- H/RConn1
  Controlled Voltage Source/LConn1 -- Voltage Sensor/RConn2 -- Lithium Cell 1RC/LConn2
  N-1/LConn1 -- Voltage Sensor/RConn1
  Voltage Sensor/LConn1 -- Lithium Cell 1RC/RConn3 -- +/RConn1
  N-1/RConn1 -- Controlled Voltage Source/RConn1
  Controlled Voltage Source/RConn2 -- -/RConn1

== system EvReferenceApplication/Passenger Car/Electric Plant/Powertrain Blockset/Battery Cooling/Battery1/Pack 2 ==
  note: Scale up voltage drop
      | to total of N cells
  Controlled Voltage Source : fl_lib/Electrical/Electrical Sources/Controlled Voltage Source
  Lithium Cell 1RC : Subsystem  Tag=PublishSubsystem
      mask Display:
      | % Battery icon
      | plot([0 0 0.8 0.8],[0.2 0.9 0.9 1.5])
      | plot([0 0 0.8 0.8],-[0.2 0.9 0.9 1.5])
      | patch([-0.4 0.4 0.4 -0.4],[-0.45 -0.45 -0.15 -0.15],[0;0;0]);
      | patch([-0.9 0.9 0.9 -0.9],[0.15 0.15 0.45 0.45],[0;0;0]);
      | 
      | % Plot points to set plot range
      | color('white');plot(1.5,1.5);plot(-1.5,-1.5)
      | 
      | color('red')
      | port_label('RConn',1,'P')
      | port_label('RConn',2,'+')
      | port_label('LConn',1,'T')
      | port_label('LConn',2,'-')
  N : fl_lib/Physical Signals/Functions/PS Gain  gain=Ncells
  N-1 : fl_lib/Physical Signals/Functions/PS Gain  gain=(Ncells-1)
  Thermal Model : Subsystem
  Voltage Sensor : fl_lib/Electrical/Electrical Sensors/Voltage Sensor
  - : PMIOPort  Tag=PMCPort  Side=Right
  H : PMIOPort  Tag=PMCPort  Port=2  Side=Left
  + : PMIOPort  Tag=PMCPort  Port=3  Side=Left
  SOC : PMIOPort  Port=4  Side=Right
  T : PMIOPort  Port=5  Side=Right
  connections:
  Controlled Voltage Source/RConn2 -- -/RConn1
  N-1/RConn1 -- Controlled Voltage Source/RConn1
  +/RConn1 -- Lithium Cell 1RC/RConn3 -- Voltage Sensor/LConn1
  N-1/LConn1 -- Voltage Sensor/RConn1
  Lithium Cell 1RC/LConn2 -- Voltage Sensor/RConn2 -- Controlled Voltage Source/LConn1
  Thermal Model/LConn1 -- H/RConn1
  Thermal Model/RConn1 -- T/RConn1 -- Lithium Cell 1RC/LConn1
  N/LConn1 -- Lithium Cell 1RC/RConn1
  N/RConn1 -- Thermal Model/LConn2
  SOC/RConn1 -- Lithium Cell 1RC/RConn2

== system EvReferenceApplication/Passenger Car/Electric Plant/Powertrain Blockset/Battery Cooling/Battery1/Pack 3 ==
  note: Scale up voltage drop
      | to total of N cells
  Controlled Voltage Source : fl_lib/Electrical/Electrical Sources/Controlled Voltage Source
  Lithium Cell 1RC : Subsystem  Tag=PublishSubsystem
      mask Display:
      | % Battery icon
      | plot([0 0 0.8 0.8],[0.2 0.9 0.9 1.5])
      | plot([0 0 0.8 0.8],-[0.2 0.9 0.9 1.5])
      | patch([-0.4 0.4 0.4 -0.4],[-0.45 -0.45 -0.15 -0.15],[0;0;0]);
      | patch([-0.9 0.9 0.9 -0.9],[0.15 0.15 0.45 0.45],[0;0;0]);
      | 
      | % Plot points to set plot range
      | color('white');plot(1.5,1.5);plot(-1.5,-1.5)
      | 
      | color('red')
      | port_label('RConn',1,'P')
      | port_label('RConn',2,'+')
      | port_label('LConn',1,'T')
      | port_label('LConn',2,'-')
  N : fl_lib/Physical Signals/Functions/PS Gain  gain=Ncells
  N-1 : fl_lib/Physical Signals/Functions/PS Gain  gain=(Ncells-1)
  Thermal Model : Subsystem
  Voltage Sensor : fl_lib/Electrical/Electrical Sensors/Voltage Sensor
  - : PMIOPort  Tag=PMCPort  Side=Right
  H : PMIOPort  Tag=PMCPort  Port=2  Side=Left
  + : PMIOPort  Tag=PMCPort  Port=3  Side=Left
  SOC : PMIOPort  Port=4  Side=Right
  T : PMIOPort  Port=5  Side=Right
  connections:
  SOC/RConn1 -- Lithium Cell 1RC/RConn2
  N/RConn1 -- Thermal Model/LConn2
  N/LConn1 -- Lithium Cell 1RC/RConn1
  Lithium Cell 1RC/LConn1 -- T/RConn1 -- Thermal Model/RConn1
  Thermal Model/LConn1 -- H/RConn1
  Controlled Voltage Source/LConn1 -- Voltage Sensor/RConn2 -- Lithium Cell 1RC/LConn2
  N-1/LConn1 -- Voltage Sensor/RConn1
  Voltage Sensor/LConn1 -- Lithium Cell 1RC/RConn3 -- +/RConn1
  N-1/RConn1 -- Controlled Voltage Source/RConn1
  Controlled Voltage Source/RConn2 -- -/RConn1

== system EvReferenceApplication/Passenger Car/Electric Plant/Powertrain Blockset/Battery Cooling/Battery1/Pack 4 ==
  note: Scale up voltage drop
      | to total of N cells
  Controlled Voltage Source : fl_lib/Electrical/Electrical Sources/Controlled Voltage Source
  Lithium Cell 1RC : Subsystem  Tag=PublishSubsystem
      mask Display:
      | % Battery icon
      | plot([0 0 0.8 0.8],[0.2 0.9 0.9 1.5])
      | plot([0 0 0.8 0.8],-[0.2 0.9 0.9 1.5])
      | patch([-0.4 0.4 0.4 -0.4],[-0.45 -0.45 -0.15 -0.15],[0;0;0]);
      | patch([-0.9 0.9 0.9 -0.9],[0.15 0.15 0.45 0.45],[0;0;0]);
      | 
      | % Plot points to set plot range
      | color('white');plot(1.5,1.5);plot(-1.5,-1.5)
      | 
      | color('red')
      | port_label('RConn',1,'P')
      | port_label('RConn',2,'+')
      | port_label('LConn',1,'T')
      | port_label('LConn',2,'-')
  N : fl_lib/Physical Signals/Functions/PS Gain  gain=Ncells
  N-1 : fl_lib/Physical Signals/Functions/PS Gain  gain=(Ncells-1)
  Thermal Model : Subsystem
  Voltage Sensor : fl_lib/Electrical/Electrical Sensors/Voltage Sensor
  - : PMIOPort  Tag=PMCPort  Side=Right
  H : PMIOPort  Tag=PMCPort  Port=2  Side=Left
  + : PMIOPort  Tag=PMCPort  Port=3  Side=Left
  SOC : PMIOPort  Port=4  Side=Right
  T : PMIOPort  Port=5  Side=Right
  connections:
  Controlled Voltage Source/RConn2 -- -/RConn1
  N-1/RConn1 -- Controlled Voltage Source/RConn1
  +/RConn1 -- Lithium Cell 1RC/RConn3 -- Voltage Sensor/LConn1
  N-1/LConn1 -- Voltage Sensor/RConn1
  Lithium Cell 1RC/LConn2 -- Voltage Sensor/RConn2 -- Controlled Voltage Source/LConn1
  Thermal Model/LConn1 -- H/RConn1
  Thermal Model/RConn1 -- T/RConn1 -- Lithium Cell 1RC/LConn1
  N/LConn1 -- Lithium Cell 1RC/RConn1
  N/RConn1 -- Thermal Model/LConn2
  SOC/RConn1 -- Lithium Cell 1RC/RConn2

== system EvReferenceApplication/Passenger Car/Electric Plant/Powertrain Blockset/Battery Cooling/Battery1/Voltage Sensor ==
  Voltage Sensor : fl_lib/Electrical/Electrical Sensors/Voltage Sensor
  + : PMIOPort  Side=Left
  - : PMIOPort  Port=2  Side=Right
  connections:
  -/RConn1 -- Voltage Sensor/RConn2
  +/RConn1 -- Voltage Sensor/LConn1

== system EvReferenceApplication/Passenger Car/Electric Plant/Powertrain Blockset/Battery Cooling/Cold Plate/Cooling Plate (Pack 1) ==
  Battery to plate conduction left : fl_lib/Thermal/Thermal Elements/Conductive Heat Transfer  thermal_type=foundation.enum.ConstantVariableTabulated.Constant  wall_geometry=foundation.enum.ConductionWallGeometry.Planar  area=0.5 m^2  thickness=1 mm  d_in=0.05 m  d_out=0.1 m  L=1 m  th_cond_min=10 W/(K*m)  th_cond=205 W/(m*K)  th_cond_TLU=[413, 401, 392, 383, 371, 357, 342] W/(K*m)  temp_TLU=[200, 273, 400, 600, 800, 1000, 1200] K  T_specify=off  T_priority=None  T=0 K  T_nominal_specify=off  T_nominal_unit=K  T_nominal_value=1  Q_specify=off  Q_priority=None  Q=0 W  Q_nominal_specify=off  Q_nominal_unit=W  Q_nominal_value=1
  "Battery to plate conduction right " : fl_lib/Thermal/Thermal Elements/Conductive Heat Transfer  thermal_type=foundation.enum.ConstantVariableTabulated.Constant  wall_geometry=foundation.enum.ConductionWallGeometry.Planar  area=0.5 m^2  thickness=1 mm  d_in=0.05 m  d_out=0.1 m  L=1 m  th_cond_min=10 W/(K*m)  th_cond=205 W/(m*K)  th_cond_TLU=[413, 401, 392, 383, 371, 357, 342] W/(K*m)  temp_TLU=[200, 273, 400, 600, 800, 1000, 1200] K  T_specify=off  T_priority=None  T=0 K  T_nominal_specify=off  T_nominal_unit=K  T_nominal_value=1  Q_specify=off  Q_priority=None  Q=0 W  Q_nominal_specify=off  Q_nominal_unit=W  Q_nominal_value=1
  Cooling channels conduction : fl_lib/Thermal/Thermal Elements/Conductive Heat Transfer  thermal_type=foundation.enum.ConstantVariableTabulated.Constant  wall_geometry=foundation.enum.ConductionWallGeometry.Planar  area=1000*0.5 cm^2  thickness=6 cm  d_in=0.05 m  d_out=0.1 m  L=1 m  th_cond_min=10 W/(K*m)  th_cond=205 W/(m*K)  th_cond_TLU=[413, 401, 392, 383, 371, 357, 342] W/(K*m)  temp_TLU=[200, 273, 400, 600, 800, 1000, 1200] K  T_specify=off  T_priority=None  T=0 K  T_nominal_specify=off  T_nominal_unit=K  T_nominal_value=1  Q_specify=off  Q_priority=None  Q=0 W  Q_nominal_specify=off  Q_nominal_unit=W  Q_nominal_value=1
  "Plate mass left " : fl_lib/Thermal/Thermal Elements/Thermal Mass  mass_type=foundation.enum.constant_variable.constant  mass=10 kg  sp_heat=910 J/kg/K  mass_min=1e-6 kg  num_ports=foundation.enum.numPorts2.one  m_specify=off  m_priority=High  m=1 kg  m_nominal_specify=off  m_nominal_unit=kg  m_nominal_value=1  T_specify=on  T_priority=High  T=bat_temp_init+273.15 K  T_nominal_specify=off  T_nominal_unit=K  T_nominal_value=1  Q_specify=off  Q_priority=None  Q=0 W  Q_nominal_specify=off  Q_nominal_unit=W  Q_nominal_value=1
  Plate mass right : fl_lib/Thermal/Thermal Elements/Thermal Mass  mass_type=foundation.enum.constant_variable.constant  mass=10 kg  sp_heat=910 J/kg/K  mass_min=1e-6 kg  num_ports=foundation.enum.numPorts2.one  m_specify=off  m_priority=High  m=1 kg  m_nominal_specify=off  m_nominal_unit=kg  m_nominal_value=1  T_specify=on  T_priority=High  T=bat_temp_init+273.15 K  T_nominal_specify=off  T_nominal_unit=K  T_nominal_value=1  Q_specify=off  Q_priority=None  Q=0 W  Q_nominal_specify=off  Q_nominal_unit=W  Q_nominal_value=1
  H1 : PMIOPort  Side=Left
  H2 : PMIOPort  Port=2  Side=Right
  T1 : PMIOPort  Port=3  Side=Left
  connections:
  Plate mass right/LConn1 -- Cooling channels conduction/RConn1 -- H2/RConn1 -- "Battery to plate conduction right "/RConn1
  T1/RConn1 -- Battery to plate conduction left/LConn1 -- "Battery to plate conduction right "/LConn1
  Battery to plate conduction left/RConn1 -- Cooling channels conduction/LConn1 -- H1/RConn1 -- "Plate mass left "/LConn1

== system EvReferenceApplication/Passenger Car/Electric Plant/Powertrain Blockset/Battery Cooling/Cold Plate/Cooling Plate (Pack 2) ==
  Battery to plate conduction left : fl_lib/Thermal/Thermal Elements/Conductive Heat Transfer  thermal_type=foundation.enum.ConstantVariableTabulated.Constant  wall_geometry=foundation.enum.ConductionWallGeometry.Planar  area=0.5 m^2  thickness=1 mm  d_in=0.05 m  d_out=0.1 m  L=1 m  th_cond_min=10 W/(K*m)  th_cond=205 W/(m*K)  th_cond_TLU=[413, 401, 392, 383, 371, 357, 342] W/(K*m)  temp_TLU=[200, 273, 400, 600, 800, 1000, 1200] K  T_specify=off  T_priority=None  T=0 K  T_nominal_specify=off  T_nominal_unit=K  T_nominal_value=1  Q_specify=off  Q_priority=None  Q=0 W  Q_nominal_specify=off  Q_nominal_unit=W  Q_nominal_value=1
  "Battery to plate conduction right " : fl_lib/Thermal/Thermal Elements/Conductive Heat Transfer  thermal_type=foundation.enum.ConstantVariableTabulated.Constant  wall_geometry=foundation.enum.ConductionWallGeometry.Planar  area=0.5 m^2  thickness=1 mm  d_in=0.05 m  d_out=0.1 m  L=1 m  th_cond_min=10 W/(K*m)  th_cond=205 W/(m*K)  th_cond_TLU=[413, 401, 392, 383, 371, 357, 342] W/(K*m)  temp_TLU=[200, 273, 400, 600, 800, 1000, 1200] K  T_specify=off  T_priority=None  T=0 K  T_nominal_specify=off  T_nominal_unit=K  T_nominal_value=1  Q_specify=off  Q_priority=None  Q=0 W  Q_nominal_specify=off  Q_nominal_unit=W  Q_nominal_value=1
  Cooling channels conduction : fl_lib/Thermal/Thermal Elements/Conductive Heat Transfer  thermal_type=foundation.enum.ConstantVariableTabulated.Constant  wall_geometry=foundation.enum.ConductionWallGeometry.Planar  area=1000*0.5 cm^2  thickness=6 cm  d_in=0.05 m  d_out=0.1 m  L=1 m  th_cond_min=10 W/(K*m)  th_cond=205 W/(m*K)  th_cond_TLU=[413, 401, 392, 383, 371, 357, 342] W/(K*m)  temp_TLU=[200, 273, 400, 600, 800, 1000, 1200] K  T_specify=off  T_priority=None  T=0 K  T_nominal_specify=off  T_nominal_unit=K  T_nominal_value=1  Q_specify=off  Q_priority=None  Q=0 W  Q_nominal_specify=off  Q_nominal_unit=W  Q_nominal_value=1
  "Plate mass left " : fl_lib/Thermal/Thermal Elements/Thermal Mass  mass_type=foundation.enum.constant_variable.constant  mass=10 kg  sp_heat=910 J/kg/K  mass_min=1e-6 kg  num_ports=foundation.enum.numPorts2.one  m_specify=off  m_priority=High  m=1 kg  m_nominal_specify=off  m_nominal_unit=kg  m_nominal_value=1  T_specify=on  T_priority=High  T=bat_temp_init+273.15 K  T_nominal_specify=off  T_nominal_unit=K  T_nominal_value=1  Q_specify=off  Q_priority=None  Q=0 W  Q_nominal_specify=off  Q_nominal_unit=W  Q_nominal_value=1
  Plate mass right : fl_lib/Thermal/Thermal Elements/Thermal Mass  mass_type=foundation.enum.constant_variable.constant  mass=10 kg  sp_heat=910 J/kg/K  mass_min=1e-6 kg  num_ports=foundation.enum.numPorts2.one  m_specify=off  m_priority=High  m=1 kg  m_nominal_specify=off  m_nominal_unit=kg  m_nominal_value=1  T_specify=on  T_priority=High  T=bat_temp_init+273.15 K  T_nominal_specify=off  T_nominal_unit=K  T_nominal_value=1  Q_specify=off  Q_priority=None  Q=0 W  Q_nominal_specify=off  Q_nominal_unit=W  Q_nominal_value=1
  H1 : PMIOPort  Side=Left
  H2 : PMIOPort  Port=2  Side=Right
  T2 : PMIOPort  Port=3  Side=Left
  connections:
  H1/RConn1 -- "Plate mass left "/LConn1 -- Battery to plate conduction left/RConn1 -- Cooling channels conduction/LConn1
  "Battery to plate conduction right "/LConn1 -- T2/RConn1 -- Battery to plate conduction left/LConn1
  Cooling channels conduction/RConn1 -- "Battery to plate conduction right "/RConn1 -- Plate mass right/LConn1 -- H2/RConn1

== system EvReferenceApplication/Passenger Car/Electric Plant/Powertrain Blockset/Battery Cooling/Cold Plate/Cooling Plate (Pack 3) ==
  Battery to plate conduction left : fl_lib/Thermal/Thermal Elements/Conductive Heat Transfer  thermal_type=foundation.enum.ConstantVariableTabulated.Constant  wall_geometry=foundation.enum.ConductionWallGeometry.Planar  area=0.5 m^2  thickness=1 mm  d_in=0.05 m  d_out=0.1 m  L=1 m  th_cond_min=10 W/(K*m)  th_cond=205 W/(m*K)  th_cond_TLU=[413, 401, 392, 383, 371, 357, 342] W/(K*m)  temp_TLU=[200, 273, 400, 600, 800, 1000, 1200] K  T_specify=off  T_priority=None  T=0 K  T_nominal_specify=off  T_nominal_unit=K  T_nominal_value=1  Q_specify=off  Q_priority=None  Q=0 W  Q_nominal_specify=off  Q_nominal_unit=W  Q_nominal_value=1
  "Battery to plate conduction right " : fl_lib/Thermal/Thermal Elements/Conductive Heat Transfer  thermal_type=foundation.enum.ConstantVariableTabulated.Constant  wall_geometry=foundation.enum.ConductionWallGeometry.Planar  area=0.5 m^2  thickness=1 mm  d_in=0.05 m  d_out=0.1 m  L=1 m  th_cond_min=10 W/(K*m)  th_cond=205 W/(m*K)  th_cond_TLU=[413, 401, 392, 383, 371, 357, 342] W/(K*m)  temp_TLU=[200, 273, 400, 600, 800, 1000, 1200] K  T_specify=off  T_priority=None  T=0 K  T_nominal_specify=off  T_nominal_unit=K  T_nominal_value=1  Q_specify=off  Q_priority=None  Q=0 W  Q_nominal_specify=off  Q_nominal_unit=W  Q_nominal_value=1
  Cooling channels conduction : fl_lib/Thermal/Thermal Elements/Conductive Heat Transfer  thermal_type=foundation.enum.ConstantVariableTabulated.Constant  wall_geometry=foundation.enum.ConductionWallGeometry.Planar  area=1000*0.5 cm^2  thickness=6 cm  d_in=0.05 m  d_out=0.1 m  L=1 m  th_cond_min=10 W/(K*m)  th_cond=205 W/(m*K)  th_cond_TLU=[413, 401, 392, 383, 371, 357, 342] W/(K*m)  temp_TLU=[200, 273, 400, 600, 800, 1000, 1200] K  T_specify=off  T_priority=None  T=0 K  T_nominal_specify=off  T_nominal_unit=K  T_nominal_value=1  Q_specify=off  Q_priority=None  Q=0 W  Q_nominal_specify=off  Q_nominal_unit=W  Q_nominal_value=1
  "Plate mass left " : fl_lib/Thermal/Thermal Elements/Thermal Mass  mass_type=foundation.enum.constant_variable.constant  mass=10 kg  sp_heat=910 J/kg/K  mass_min=1e-6 kg  num_ports=foundation.enum.numPorts2.one  m_specify=off  m_priority=High  m=1 kg  m_nominal_specify=off  m_nominal_unit=kg  m_nominal_value=1  T_specify=on  T_priority=High  T=bat_temp_init+273.15 K  T_nominal_specify=off  T_nominal_unit=K  T_nominal_value=1  Q_specify=off  Q_priority=None  Q=0 W  Q_nominal_specify=off  Q_nominal_unit=W  Q_nominal_value=1
  Plate mass right : fl_lib/Thermal/Thermal Elements/Thermal Mass  mass_type=foundation.enum.constant_variable.constant  mass=10 kg  sp_heat=910 J/kg/K  mass_min=1e-6 kg  num_ports=foundation.enum.numPorts2.one  m_specify=off  m_priority=High  m=1 kg  m_nominal_specify=off  m_nominal_unit=kg  m_nominal_value=1  T_specify=on  T_priority=High  T=bat_temp_init+273.15 K  T_nominal_specify=off  T_nominal_unit=K  T_nominal_value=1  Q_specify=off  Q_priority=None  Q=0 W  Q_nominal_specify=off  Q_nominal_unit=W  Q_nominal_value=1
  H1 : PMIOPort  Side=Left
  H2 : PMIOPort  Port=2  Side=Right
  T3 : PMIOPort  Port=3  Side=Left
  connections:
  "Plate mass left "/LConn1 -- H1/RConn1 -- Cooling channels conduction/LConn1 -- Battery to plate conduction left/RConn1
  "Battery to plate conduction right "/LConn1 -- Battery to plate conduction left/LConn1 -- T3/RConn1
  "Battery to plate conduction right "/RConn1 -- H2/RConn1 -- Cooling channels conduction/RConn1 -- Plate mass right/LConn1
